simulink model "may9js"  (R2015a)
settings: Solver=ode4  StartTime=0.0  StopTime=inf  FixedStep=BKIN_STEP_TIME  RelTol=1e-3
StartFcn:
  |  warndlg('Dexterit-E models cannot run under simulation. Please compile your model and run it from within Dexterit-E.');set_param(bdroot,'SimulationCommand','stop')
model workspace (MAT data in the model file):
  BARRIER_ROW = 5
  BKIN_KINEMATIC_FRAME_SIZE = 400
  BKIN_STEP_TIME = 0.00025
  CIRCLE_ROW = 2
  CIRCLE_STROKE = 10
  CIRCLE_STROKE_W = 11
  E_BARRIER_HIT = 6
  E_COLLISION_HIT = 7
  E_ENTER_PRESHOT_AREA = 2
  E_ENTER_START_AREA = 12
  E_EXIT = 13
  E_EXIT_PRESHOT_AREA = 10
  E_GOAL_HIT = 8
  E_GOAL_REACHED = 5
  E_NO_EVENT = 0
  E_PRESHOT_ROW = 4
  E_TARGET_OUT_OF_BOUNDS = 9
  E_TRIAL_BEGIN = 1
  E_TRIAL_ENDED = 3
  FIRST_STATE_FILL = 9
  FORCE_MULTIPLIER = 1
  F_BUMP = 1
  GOAL_ROW = 8
  GOAL_TIME = 15
  HEIGHT = 6
  INVISIBLE_FILL = 15
  LOAD_ROW = 4
  MASS_BARRIER = 6
  MASS_CIRCLE = 2
  MASS_RECT = 3
  NEW_FLOAT = 10
  NEW_ROW = 9
  NEW_TEXTSIZE = 11
  PERT_DUR = 5
  PERT_RAMP = 4
  PRESHOT_ROW = 7
  RADIUS_LOG = 4
  RADIUS_VIS = 5
  RECT_FILL = 12
  RECT_ROW = 3
  RECT_STROKE = 13
  RECT_STROKE_W = 14
  ROTATION = 7
  SECONDS = 1
  SECOND_STATE_FILL = 8
  SHOT_READY_TIME = 13
  SHOT_SET_TIME = 14
  START_HOLD_TIME = 12
  START_ROW = 6
  TRIAL_FAILURE = 11
  WIDTH = 3
  col_x = 1
  col_y = 2
undefined symbols (not defined in the file): slselsubs
libraries: Video x7, General x3, KINARM_loads x2, KINARM_EP_loads x1, KINARM_general x1, simulink x1, slrtlib x1
(part 3 of 4)

== stateflow chart may9js/subsystem for moving the square (updating velocity and checking collision)/Collision Resolution ==
  settings: sampleTime=0.001
  state Initialize/
    % Stateflow starts here when task is loaded
    entry: force_scaling = [0 0 0 0];
    rect_target_out = zeros(1,70);
    rect_vel = [0 0];
    rect_offset_position = [0 0];
    trial_step = 0;
    trial_stop = 0;
  state Initialize1/
    % Stateflow starts here when task is loaded
    entry: force_scaling = [0 0 0 0];
    rect_target_out = zeros(1,70);
    rect_vel = [0 0];
    rect_offset_position = [0 0];
    trial_step = 0;
    trial_stop = 0;
  state Moving_Targets_and_Colliding_Them
    %there are 4 parallel states here. They each execute in the same cycle but in a specific order (see top right of the state)
    % state 3 is the important one - it simply says "move the square according to its velocity"
    % states 1 and 2 check collisions to update that velocity before we get to state 3
    % state 4 then checks to see if we ended up outside the screen and if so, to take us back to the start position
    state CollisionWithWall/ [parallel] [commented out]
      % this substate will handle collision between square and screen edges.
      % is the rectangle at the left edge of the screen
      en, du: if((rect_target_out(3)-rect_target_out(10)/2) < -display_size(1)/2)
      %rect_vel(1) = -rect_vel(1);
      trial_step = 2
      rect_vel(1) = 0;
      end
      % is the rectangle at the right edge of the screen
      if((rect_target_out(3)+rect_target_out(10)/2) > display_size(1)/2)
      %rect_vel(1) = -rect_vel(1);
      trial_step = 2
      rect_vel(1) = 0;
      end
      % is the rectangle at top of the scren
      if((rect_target_out(4)+rect_target_out(11)/2) > display_size(2))
      %rect_vel(2) = -rect_vel(2);
      trial_step = 2
      rect_vel(2) = 0;
      end
      % is the rectangle at bottom of the scren
      if((rect_target_out(4)-rect_target_out(11)/2) < 0)
      trial_step = 2
      rect_vel(2) = 0;
      %rect_vel(2) = -rect_vel(2);
      end
    state CheckToSeeIfWeAreOutofBounds1/ [parallel] [commented out]
      % once everything is done moving and colliding, we check to see if we're off the screen still. If we are, put the square in the start position with 0 velocity
      % once collision is handled, move the square by its velocity
      % Reset everything as soon as the rectangle touches the side of the screen
      during:
      if (rect_target_out(3) - rect_target_out(10)/2 <= -display_size(1)/2) || ...
      (rect_target_out(3) + rect_target_out(10)/2 >= display_size(1)/2) || ...
      (rect_target_out(4) + rect_target_out(11)/2 >= display_size(2)) || ...
      (rect_target_out(4) - rect_target_out(11)/2 <= 0)
      % Reset all movement variables
      rect_vel = [0, 0];  % Stop movement
      rect_offset_position = [0, 0];  % Reset position
      trial_step = 4;
      trial_stop = 1;  % Set flag to stop trial
      end
    state CheckToSeeIfGoalReached1/ [parallel] [commented out]
      % once the participant hits the square (denoted by the puck), then we want to calculate if it is inside of the goal or not. this is done using the input form prior matrix.
      % since the input ot this block is the vcode, we access the dimesnion of the vector that contains length., width, height. in the start position with 0 velocity
      % Get rectangle (puck) info
      rect_x = rect_target_out(3);
      rect_y = rect_target_out(4);
      rect_w = rect_target_out(10);
      rect_h = rect_target_out(11);
      % Get goal info
      goal_x = goal_target(3);
      goal_y = goal_target(4);
      goal_w = goal_target(10);
      goal_h = goal_target(11);
      % Compute edges
      rect_left   = rect_x - rect_w / 2;
      rect_right  = rect_x + rect_w / 2;
      rect_top    = rect_y + rect_h / 2;
      rect_bottom = rect_y - rect_h / 2;
      goal_left   = goal_x - goal_w / 2;
      goal_right  = goal_x + goal_w / 2;
      goal_top    = goal_y + goal_h / 2;
      goal_bottom = goal_y - goal_h / 2;
      % Check for full puck in goal (fully inside goal)
      if (rect_left >= goal_left) && (rect_right <= goal_right) && ...
      (rect_bottom >= goal_bottom) && (rect_top <= goal_top)
      % Fully inside goal
      trial_step = 3;
      trial_stop = 1;
      %rect_vel = [0, 0];  % Stop motion
      %rect_offset_position = [0, 0];  % Optionalreset
      end
    state CollisionWithHand/ [parallel]
      % this substate will handle collision checks between hands and the square
      settings: executionOrder=1
      state ResolveTargetCollision
        during: % if something collided, we're going to separate the two objects and then use elastic collision to update velocities
        % eject the rectangle
        rect_offset_position = eject( circ_target( target_colliding,:), rect_target, rect_offset_position);
        prev_vel = rect_vel;
        hand_vel = hand_speed( target_colliding,:)/1e3;
        % elastic collision equations - here m = 1 and is the same for hand and square. It is used here to provide relative mass
        % between the two objects. The forces here will be further multiplied by a fudge factor (see the Simulink forces section)
        rect_vel(1) = (mr - mc)/(mr + mc)*rect_vel(1) + 2*mc/(mc + mr)*hand_vel(1);
        rect_vel(2) = (mr - mc)/(mr + mc)*rect_vel(2) + 2*mc/(mc + mr)*hand_vel(2);
        hand_vector = [1 2; 3 4];
        % a bump will be generated that will be proportional to change in velocity
        force_scaling(hand_vector(target_colliding,:)) = prev_vel - rect_vel;
      state WaitForCollision/
        entry: % state where we wait for collisions to happen
        force_scaling = [0 0 0 0];
        during:
        rect_target_out = rect_target;
        rect_offset_position = rect_offset_position + rect_vel;
        rect_target_out(3:4) = rect_target_out(3:4)+rect_offset_position
        target_colliding = check_collision(circ_target, rect_target, rect_offset_position)
      state StartWithSpeed0/
        %
        entry:  rect_vel = [0 0];
        rect_offset_position = [0 0];
      Moving_Targets_and_Colliding_Them.CollisionWithHand.WaitForCollision -> Moving_Targets_and_Colliding_Them.CollisionWithHand.StartWithSpeed0 [order 2] : e_Trial_Start
      Moving_Targets_and_Colliding_Them.CollisionWithHand.StartWithSpeed0 -> Moving_Targets_and_Colliding_Them.CollisionWithHand.WaitForCollision
      Moving_Targets_and_Colliding_Them.CollisionWithHand.WaitForCollision -> Moving_Targets_and_Colliding_Them.CollisionWithHand.ResolveTargetCollision [order 1] : [ target_colliding]
      Moving_Targets_and_Colliding_Them.CollisionWithHand.ResolveTargetCollision -> Moving_Targets_and_Colliding_Them.CollisionWithHand.WaitForCollision : [~check_collision(circ_target( target_colliding,:), rect_target, rect_offset_position)]
          | /{target_colliding=0}
    state PositionUpdated/ [parallel]
      % once collision is handled, move the square by its velocity
      during: rect_target_out = rect_target;
      rect_offset_position = rect_offset_position + rect_vel;
      rect_target_out(3:4) = rect_target_out(3:4)+rect_offset_position;
      settings: executionOrder=2
  state Moving_Targets_and_Colliding_Them1
    %there are 4 parallel states here. They each execute in the same cycle but in a specific order (see top right of the state)
    % state 3 is the important one - it simply says "move the square according to its velocity"
    % states 1 and 2 check collisions to update that velocity before we get to state 3
    % state 4 then checks to see if we ended up outside the screen and if so, to take us back to the start position
    state PositionUpdated/ [parallel]
      % once collision is handled, move the square by its velocity
      during: rect_target_out = rect_target;
      rect_offset_position = rect_offset_position + rect_vel;
      rect_target_out(3:4) = rect_target_out(3:4)+rect_offset_position;
      settings: executionOrder=2
    state CollisionWithHand/ [parallel]
      % this substate will handle collision checks between hands and the square
      settings: executionOrder=1
      state StartWithSpeed0/
        %
        entry:  rect_vel = [0 0];
        rect_offset_position = [0 0];
      state WaitForCollision/
        entry: % state where we wait for collisions to happen
        force_scaling = [0 0 0 0];
        during:
        rect_target_out = rect_target;
        rect_offset_position = rect_offset_position + rect_vel;
        rect_target_out(3:4) = rect_target_out(3:4)+rect_offset_position
        target_colliding = check_collision(circ_target, rect_target, rect_offset_position)
      state ResolveTargetCollision
        during: % if something collided, we're going to separate the two objects and then use elastic collision to update velocities
        % eject the rectangle
        rect_offset_position = eject( circ_target( target_colliding,:), rect_target, rect_offset_position);
        prev_vel = rect_vel;
        hand_vel = hand_speed( target_colliding,:)/1e3;
        % elastic collision equations - here m = 1 and is the same for hand and square. It is used here to provide relative mass
        % between the two objects. The forces here will be further multiplied by a fudge factor (see the Simulink forces section)
        rect_vel(1) = (mr - mc)/(mr + mc)*rect_vel(1) + 2*mc/(mc + mr)*hand_vel(1);
        rect_vel(2) = (mr - mc)/(mr + mc)*rect_vel(2) + 2*mc/(mc + mr)*hand_vel(2);
        hand_vector = [1 2; 3 4];
        % a bump will be generated that will be proportional to change in velocity
        force_scaling(hand_vector(target_colliding,:)) = prev_vel - rect_vel;
      Moving_Targets_and_Colliding_Them1.CollisionWithHand.WaitForCollision -> Moving_Targets_and_Colliding_Them1.CollisionWithHand.StartWithSpeed0 [order 2] : e_Trial_Start
      Moving_Targets_and_Colliding_Them1.CollisionWithHand.StartWithSpeed0 -> Moving_Targets_and_Colliding_Them1.CollisionWithHand.WaitForCollision
      Moving_Targets_and_Colliding_Them1.CollisionWithHand.WaitForCollision -> Moving_Targets_and_Colliding_Them1.CollisionWithHand.ResolveTargetCollision [order 1] : [ target_colliding]
      Moving_Targets_and_Colliding_Them1.CollisionWithHand.ResolveTargetCollision -> Moving_Targets_and_Colliding_Them1.CollisionWithHand.WaitForCollision : [~check_collision(circ_target( target_colliding,:), rect_target, rect_offset_position)]
          | /{target_colliding=0}
    state CheckToSeeIfGoalReached1/ [parallel] [commented out]
      % once the participant hits the square (denoted by the puck), then we want to calculate if it is inside of the goal or not. this is done using the input form prior matrix.
      % since the input ot this block is the vcode, we access the dimesnion of the vector that contains length., width, height. in the start position with 0 velocity
      % Get rectangle (puck) info
      rect_x = rect_target_out(3);
      rect_y = rect_target_out(4);
      rect_w = rect_target_out(10);
      rect_h = rect_target_out(11);
      % Get goal info
      goal_x = goal_target(3);
      goal_y = goal_target(4);
      goal_w = goal_target(10);
      goal_h = goal_target(11);
      % Compute edges
      rect_left   = rect_x - rect_w / 2;
      rect_right  = rect_x + rect_w / 2;
      rect_top    = rect_y + rect_h / 2;
      rect_bottom = rect_y - rect_h / 2;
      goal_left   = goal_x - goal_w / 2;
      goal_right  = goal_x + goal_w / 2;
      goal_top    = goal_y + goal_h / 2;
      goal_bottom = goal_y - goal_h / 2;
      % Check for full puck in goal (fully inside goal)
      if (rect_left >= goal_left) && (rect_right <= goal_right) && ...
      (rect_bottom >= goal_bottom) && (rect_top <= goal_top)
      % Fully inside goal
      trial_step = 3;
      trial_stop = 1;
      %rect_vel = [0, 0];  % Stop motion
      %rect_offset_position = [0, 0];  % Optionalreset
      end
    state CheckToSeeIfWeAreOutofBounds1/ [parallel] [commented out]
      % once everything is done moving and colliding, we check to see if we're off the screen still. If we are, put the square in the start position with 0 velocity
      % once collision is handled, move the square by its velocity
      % Reset everything as soon as the rectangle touches the side of the screen
      during:
      if (rect_target_out(3) - rect_target_out(10)/2 <= -display_size(1)/2) || ...
      (rect_target_out(3) + rect_target_out(10)/2 >= display_size(1)/2) || ...
      (rect_target_out(4) + rect_target_out(11)/2 >= display_size(2)) || ...
      (rect_target_out(4) - rect_target_out(11)/2 <= 0)
      % Reset all movement variables
      rect_vel = [0, 0];  % Stop movement
      rect_offset_position = [0, 0];  % Reset position
      trial_step = 4;
      trial_stop = 1;  % Set flag to stop trial
      end
    state CollisionWithWall/ [parallel] [commented out]
      % this substate will handle collision between square and screen edges.
      % is the rectangle at the left edge of the screen
      en, du: if((rect_target_out(3)-rect_target_out(10)/2) < -display_size(1)/2)
      %rect_vel(1) = -rect_vel(1);
      trial_step = 2
      rect_vel(1) = 0;
      end
      % is the rectangle at the right edge of the screen
      if((rect_target_out(3)+rect_target_out(10)/2) > display_size(1)/2)
      %rect_vel(1) = -rect_vel(1);
      trial_step = 2
      rect_vel(1) = 0;
      end
      % is the rectangle at top of the scren
      if((rect_target_out(4)+rect_target_out(11)/2) > display_size(2))
      %rect_vel(2) = -rect_vel(2);
      trial_step = 2
      rect_vel(2) = 0;
      end
      % is the rectangle at bottom of the scren
      if((rect_target_out(4)-rect_target_out(11)/2) < 0)
      trial_step = 2
      rect_vel(2) = 0;
      %rect_vel(2) = -rect_vel(2);
      end
  (default) -> Initialize
  Initialize -> Moving_Targets_and_Colliding_Them.CollisionWithHand.StartWithSpeed0
  data: colliding_target function_output; circ_matrix_in function_input; rect_vector_in function_input; rect_offset_in function_input; colliding_target function_output; circ_matrix_in function_input; rect_vector_in function_input; rect_offset_in function_input; eject_rect_offset function_output; circ_vcode_in function_input; rect_vcode_in function_input; rect_offset function_input; eject_rect_offset function_output; circ_vcode_in function_input; rect_vcode_in function_input; rect_offset function_input; trial_protocol input; circ_target input double; circ_to_barrier_target input; rect_target_out output size=[1 70]; rect_target input; barrier_target input size=[1 70]; display_size input; force_scaling output; mc input; mr input; hand_vector local; rect_vel local; prev_vel local; target_colliding local; hand_vel local; rect_offset_position local double; trial_stop output double size=[1]; goal_target input; trial_step output; mb input size=1; barrier_colliding local; hand_speed input; check_collision_barrier1 local; barrier_vel local; force_scaling_barrier local; rect_y local; rect_w local; rect_h local; rect_x local; goal_h local; goal_y local; goal_w local; goal_x local; rect_top local; goal_top local; hand_offset_position local; prev_hand_vel local; rect_left local; rect_bottom local; goal_right local; rect_right local; goal_bottom local; goal_left local; new_hand_posistion_c local
  events: e_clk input RISING_EDGE_EVENT; e_Trial_Start input EITHER_EDGE_EVENT; e_Trial_Start1 input EITHER_EDGE_EVENT
  function colliding_target = check_collision(circ_matrix_in, rect_vector_in, rect_offset_in):
    | function colliding_target = check_collision(circ_matrix_in, rect_vector_in, rect_offset_in)
    | 
    | % calculates collision between 2 circles (ie. either hand feedback) and rectangle
    | % inputs:
    | %        circ_matrix_in - 2x70 matrix that is 2 circle vcodes
    | %        rect_vector_in - 1x70 vector that is a rectangle vcode
    | %        rect_offset_in - position offset for rect_vector_ in to calculate
    | %                         where the rectangle is
    | % outputs:
    | %        colliding_target values:
    | %              0- if nothing colliding
    | %              1- if rectangle collided with right hand
    | %              2- if rectangle colliding with left hand
    | 
    | x = 3;
    | y = 4;
    | 
    | colliding_target = 0;
    | 
    | for ii = 1:size(circ_matrix_in,1)
    | 	
    | 	current_circle_vcode = circ_matrix_in(ii,:);
    | 	
    | 	radius = current_circle_vcode(10);
    | 	w = rect_vector_in(10);
    | 	h = rect_vector_in(10);
    | 	
    | 	x0 = current_circle_vcode(x);
    | 	y0 = current_circle_vcode(y);
    | 	
    | 	X0 = rect_vector_in(x)+rect_offset_in(1);
    | 	Y0 = rect_vector_in(y)+rect_offset_in(2);
    | 	
    | 	deltax = x0-X0;
    | 	deltay = y0-Y0;
    | 	
    | 	w = rect_vector_in(10);  %width (sizes in cm in v1.4)
    | 	h = rect_vector_in(11);  %height (sizes in cm in v1.4)
    | 	
    | 	t = rect_vector_in(12)/180*pi;
    | 	
    | 	sint=sin(t);
    | 	cost=cos(t);
    | 	
    | 	xrotate=deltax.*cost + deltay.*sint;   %location of x point in rectangle's coordinate frame
    | 	yrotate=-deltax.*sint + deltay.*cost;  %location of y point in rectangle's coordinate frame
    | 		
    | 	%intarget = (abs(xrotate) < (w/2+radius)) & (abs(yrotate) < (h/2+radius));
    | 	
    | 	%--------------%
    | 	DeltaX = xrotate - max(0 - w/2, min(xrotate, 0 + w/2));
    | 	DeltaY = yrotate - max(0 - h/2, min(yrotate, 0 + h/2));
    | 	intarget = 1*(DeltaX * DeltaX + DeltaY * DeltaY) < (radius * radius);
    | 	
    | 	%--------------%
    | 	
    | 	
    | 	if intarget
    | 		colliding_target = ii;
    | 		break;
    | 	end
    | 	
    | end
  function colliding_target = check_collision1(circ_matrix_in, rect_vector_in, rect_offset_in):
    | function colliding_target = check_collision1(circ_matrix_in, rect_vector_in, rect_offset_in)
    | 
    | % calculates collision between 2 circles (ie. either hand feedback) and rectangle
    | % inputs:
    | %        circ_matrix_in - 2x70 matrix that is 2 circle vcodes
    | %        rect_vector_in - 1x70 vector that is a rectangle vcode
    | %        rect_offset_in - position offset for rect_vector_ in to calculate
    | %                         where the rectangle is
    | % outputs:
    | %        colliding_target values:
    | %              0- if nothing colliding
    | %              1- if rectangle collided with right hand
    | %              2- if rectangle colliding with left hand
    | 
    | x = 3;
    | y = 4;
    | 
    | colliding_target = 0;
    | 
    | for ii = 1:size(circ_matrix_in,1)
    | 	
    | 	current_circle_vcode = circ_matrix_in(ii,:);
    | 	
    | 	radius = current_circle_vcode(10);
    | 	w = rect_vector_in(10);
    | 	h = rect_vector_in(10);
    | 	
    | 	x0 = current_circle_vcode(x);
    | 	y0 = current_circle_vcode(y);
    | 	
    | 	X0 = rect_vector_in(x)+rect_offset_in(1);
    | 	Y0 = rect_vector_in(y)+rect_offset_in(2);
    | 	
    | 	deltax = x0-X0;
    | 	deltay = y0-Y0;
    | 	
    | 	w = rect_vector_in(10);  %width (sizes in cm in v1.4)
    | 	h = rect_vector_in(11);  %height (sizes in cm in v1.4)
    | 	
    | 	t = rect_vector_in(12)/180*pi;
    | 	
    | 	sint=sin(t);
    | 	cost=cos(t);
    | 	
    | 	xrotate=deltax.*cost + deltay.*sint;   %location of x point in rectangle's coordinate frame
    | 	yrotate=-deltax.*sint + deltay.*cost;  %location of y point in rectangle's coordinate frame
    | 		
    | 	%intarget = (abs(xrotate) < (w/2+radius)) & (abs(yrotate) < (h/2+radius));
    | 	
    | 	%--------------%
    | 	DeltaX = xrotate - max(0 - w/2, min(xrotate, 0 + w/2));
    | 	DeltaY = yrotate - max(0 - h/2, min(yrotate, 0 + h/2));
    | 	intarget = 1*(DeltaX * DeltaX + DeltaY * DeltaY) < (radius * radius);
    | 	
    | 	%--------------%
    | 	
    | 	
    | 	if intarget
    | 		colliding_target = ii;
    | 		break;
    | 	end
    | 	
    | end
  function eject_rect_offset = eject(circ_vcode_in, rect_vcode_in, rect_offset):
    | function eject_rect_offset = eject(circ_vcode_in, rect_vcode_in, rect_offset)
    | 
    | % moves the rectangle_vcode out of a circle_vcode if the two are
    | % overlapping
    | 
    | x = 3;
    | y = 4;
    | 
    | radius = circ_vcode_in(10);
    | w = rect_vcode_in(10);
    | h = rect_vcode_in(10);
    | 
    | x0 = circ_vcode_in(x);
    | y0 = circ_vcode_in(y);
    | 
    | X0 = rect_vcode_in(x)+rect_offset(1);
    | Y0 = rect_vcode_in(y)+rect_offset(2);
    | 
    | deltax = x0-X0;
    | deltay = y0-Y0;
    | 
    | w = rect_vcode_in(10);  %width (sizes in cm in v1.4)
    | h = rect_vcode_in(11);  %height (sizes in cm in v1.4)
    | 
    | t = rect_vcode_in(12)/180*pi;
    | 
    | sint=sin(t);
    | cost=cos(t);
    | 
    | xrotate=deltax.*cost + deltay.*sint;   %location of x point in rectangle's coordinate frame
    | yrotate=-deltax.*sint + deltay.*cost;  %location of y point in rectangle's coordinate frame
    | 
    | % so xrotate and yrotate is where the circle is inside the rectangle
    | theta_threshold = atan(h / w); % get the threshold - angles below this go out the side while angles
    | % above this go out the top
    | 
    | % calculating magnitude
    | 
    | % polar coordinate to the circle
    | [t_c, ~] = cart2pol(abs(xrotate), abs(yrotate));
    | 
    | if t_c < theta_threshold % the rectangle will be moved along its local x-axis to exit the circle
    |     x_eject_local = (w/2+radius-abs(xrotate))*sign(-xrotate); % if the circle is on the right, move the rectangle left and vice-versa
    |     y_eject_local = 0;
    | else % going out top/bottom % the rectangle will be moved along its local y-axis to exit the circle
    |     x_eject_local = 0;
    |     y_eject_local = (h/2+radius-abs(yrotate))*sign(-yrotate); % if the circle is above the rectangle, move the rectangle down and vice-versa
    | end
    | 
    | % convert the local offsets to global coordinates by undoing the rotation
    | 
    | % rotate back to global coordinates
    | sint=sin(-t);
    | cost=cos(-t);
    | 
    | x_eject_global = x_eject_local.*cost + y_eject_local.*sint;   
    | y_eject_global = - x_eject_local.*sint + y_eject_local.*cost;
    | 
    | eject_rect_offset = rect_offset + [x_eject_global y_eject_global];
  function eject_rect_offset = eject1(circ_vcode_in, rect_vcode_in, rect_offset):
    | function eject_rect_offset = eject1(circ_vcode_in, rect_vcode_in, rect_offset)
    | 
    | % moves the rectangle_vcode out of a circle_vcode if the two are
    | % overlapping
    | 
    | x = 3;
    | y = 4;
    | 
    | radius = circ_vcode_in(10);
    | w = rect_vcode_in(10);
    | h = rect_vcode_in(10);
    | 
    | x0 = circ_vcode_in(x);
    | y0 = circ_vcode_in(y);
    | 
    | X0 = rect_vcode_in(x)+rect_offset(1);
    | Y0 = rect_vcode_in(y)+rect_offset(2);
    | 
    | deltax = x0-X0;
    | deltay = y0-Y0;
    | 
    | w = rect_vcode_in(10);  %width (sizes in cm in v1.4)
    | h = rect_vcode_in(11);  %height (sizes in cm in v1.4)
    | 
    | t = rect_vcode_in(12)/180*pi;
    | 
    | sint=sin(t);
    | cost=cos(t);
    | 
    | xrotate=deltax.*cost + deltay.*sint;   %location of x point in rectangle's coordinate frame
    | yrotate=-deltax.*sint + deltay.*cost;  %location of y point in rectangle's coordinate frame
    | 
    | % so xrotate and yrotate is where the circle is inside the rectangle
    | theta_threshold = atan(h / w); % get the threshold - angles below this go out the side while angles
    | % above this go out the top
    | 
    | % calculating magnitude
    | 
    | % polar coordinate to the circle
    | [t_c, ~] = cart2pol(abs(xrotate), abs(yrotate));
    | 
    | if t_c < theta_threshold % the rectangle will be moved along its local x-axis to exit the circle
    |     x_eject_local = (w/2+radius-abs(xrotate))*sign(-xrotate); % if the circle is on the right, move the rectangle left and vice-versa
    |     y_eject_local = 0;
    | else % going out top/bottom % the rectangle will be moved along its local y-axis to exit the circle
    |     x_eject_local = 0;
    |     y_eject_local = (h/2+radius-abs(yrotate))*sign(-yrotate); % if the circle is above the rectangle, move the rectangle down and vice-versa
    | end
    | 
    | % convert the local offsets to global coordinates by undoing the rotation
    | 
    | % rotate back to global coordinates
    | sint=sin(-t);
    | cost=cos(-t);
    | 
    | x_eject_global = x_eject_local.*cost + y_eject_local.*sint;   
    | y_eject_global = - x_eject_local.*sint + y_eject_local.*cost;
    | 
    | eject_rect_offset = rect_offset + [x_eject_global y_eject_global];

== matlab function may9js/subsystem for moving the square (updating velocity and checking collision)/Hand Feedback/MATLAB Function ==
  data: feedback_vcodes input; arm_to_be_assessed input; hand_vcodes output
function hand_vcodes = fcn(feedback_vcodes, arm_to_be_assessed)
% the hand feedback vcodes are sorted like this:
%    <arm to be assessed vcode>
%    <contralateral arm> 
% but using this function I am going to sort the vcodes like this:
%    <right arm>
%    <left arm>
% because that will make it easier to track velocities and forces

if arm_to_be_assessed == 1
	hand_vcodes = feedback_vcodes;
else
	hand_vcodes = feedback_vcodes([2 1], :);
	%hand_vcodes = feedback_vcodes;
end

== stateflow chart may9js/Trial_Control ==
  settings: sampleTime=0.001
  state Initialize/
    % Set variables
    entry:
    logging_enable = true;
    start_target_row = Trial_Protocol(START_ROW);
    preshot_area_row = Trial_Protocol(PRESHOT_ROW);
    cursor_row = Trial_Protocol(CIRCLE_ROW);
    puck_row = Trial_Protocol(RECT_ROW);
    barrier_target_row = Trial_Protocol(BARRIER_ROW);
    goal_target_row = Trial_Protocol(GOAL_ROW);
    load_row = Trial_Protocol(LOAD_ROW);
    trial_duration = Trial_Protocol(SECONDS);
    start_hold_time = Trial_Protocol(START_HOLD_TIME);
    shot_ready_time = Trial_Protocol(SHOT_READY_TIME);
    shot_set_time = Trial_Protocol(SHOT_SET_TIME);
    goal_time = Trial_Protocol(GOAL_TIME);
  state Main_Trial/
    % Each trial task only initializes variables and then runs for Trial_Protocol(SECONDS) seconds before stopping
    state StartOn/
      entry:
      start_target_state = 2;
      preshot_area_state = 0;
      cursor_state = 2;
      puck_state = 0;
      barrier_target_state = 0;
      goal_target_state = 0;
      e_Trial_Start;
      event_code = E_TRIAL_BEGIN;
    state StartHold/
      entry:
      start_target_state = 3;
      preshot_area_state=0;
      puck_state=0;
      goal_target_state=0;
      barrier_target_state=0;
      event_code = E_ENTER_START_AREA;
    state PreshotStart/
      % send e_Trial_End event
      entry:
      preshot_area_state=3;
      puck_state=2;
      goal_target_state=2;
      barrier_target_state=2;
      event_code = E_ENTER_PRESHOT_AREA;
    state PreshotMove/
      % send e_Trial_End event
      entry:
    state CollisionWithHand/
      % this substate will handle collision checks between hands and the square
      state StartWithSpeed0/
        %
        entry:  rect_vel = [0 0];
        rect_offset_position = [0 0];
      state WaitForCollision/
        entry: % state where we wait for collisions to happen
        force_scaling = [0 0 0 0];
        during:
        rect_target_out = rect_target;
        rect_offset_position = rect_offset_position + rect_vel;
        rect_target_out(3:4) = rect_target_out(3:4)+rect_offset_position
        target_colliding = check_collision(circ_target, rect_target, rect_offset_position)
      state ResolveTargetCollision
        during: % if something collided, we're going to separate the two objects and then use elastic collision to update velocities
        % eject the rectangle
        rect_offset_position = eject( circ_target( target_colliding,:), rect_target, rect_offset_position);
        prev_vel = rect_vel;
        hand_vel = hand_speed( target_colliding,:)/1e3;
        % elastic collision equations - here m = 1 and is the same for hand and square. It is used here to provide relative mass
        % between the two objects. The forces here will be further multiplied by a fudge factor (see the Simulink forces section)
        rect_vel(1) = (mr - mc)/(mr + mc)*rect_vel(1) + 2*mc/(mc + mr)*hand_vel(1);
        rect_vel(2) = (mr - mc)/(mr + mc)*rect_vel(2) + 2*mc/(mc + mr)*hand_vel(2);
        hand_vector = [1 2; 3 4];
        % a bump will be generated that will be proportional to change in velocity
        force_scaling(hand_vector(target_colliding,:)) = prev_vel - rect_vel;
      WaitForCollision -> StartWithSpeed0 [order 2] : e_Trial_Start
      StartWithSpeed0 -> WaitForCollision
      WaitForCollision -> ResolveTargetCollision [order 1] : [ target_colliding]
      ResolveTargetCollision -> WaitForCollision : [~check_collision(circ_target( target_colliding,:), rect_target, rect_offset_position)]
          | /{target_colliding=0}
    state ShotReady/
      % send e_Trial_End event
      entry:
      event_code = E_EXIT;
    state ShotSet/
      % send e_Trial_End event
      entry:
      preshot_area_state=0;
    state Success/
      % send e_Trial_End event
      entry:
      puck_state=0;
      goal_target_state=3
    state PuckInGoal/
      % send e_Trial_End event
      entry:
    state Shot/
      % send e_Trial_End event
      entry:
      start_target_state=0;
    state Fail/
      % send e_Trial_End event
      entry:
      event_code = E_TRIAL_FAILURE;
      start_target_state=0;
      preshot_area_state = 0;
      cursor_state = 2;
      puck_state = 0;
      barrier_target_state = 0;
      goal_target_state = 0;
    state PositionUpdated/
      % once collision is handled, move the square by its velocity
      during: rect_target_out = rect_target;
      rect_offset_position = rect_offset_position + rect_vel;
      rect_target_out(3:4) = rect_target_out(3:4)+rect_offset_position;
    state Initialize1/
      % Stateflow starts here when task is loaded
      entry: force_scaling = [0 0 0 0];
      rect_target_out = zeros(1,70);
      rect_vel = [0 0];
      rect_offset_position = [0 0];
      trial_step = 0;
      trial_stop = 0;
    StartHold -> PreshotStart [order 2] : after(start_hold_time,sec)
    StartOn -> StartHold [order 1] : [HandInTarget(start_target_row,1)==1]
    StartHold -> StartOn [order 1] : [HandInTarget(start_target_row,1)==0]
    PreshotStart -> PreshotMove [order 2] : [HandInTarget(start_target_row,1)==0]
    PreshotStart -> StartHold [order 1] : [HandInTarget(preshot_area_row,1)==0]
    ShotSet -> StartOn [order 1] : [HandInTarget(start_target_row,1)==0]
    PreshotMove -> StartOn [order 2] : [HandInTarget(preshot_area_row,1)==0]
    ShotReady -> PreshotMove [order 1] : [HandInTarget(start_target_row,1)==0]
    PreshotMove -> ShotReady [order 1] : [HandInTarget(start_target_row,1)==1]
    ShotReady -> StartWithSpeed0 [order 2]
    ShotReady -> ShotSet [order 3] : after(shot_ready_time,sec)
    ShotSet -> Shot [order 2] : after(shot_set_time,sec)
    PuckInGoal -> Success [order 1] : after(goal_time,sec)
    Shot -> PuckInGoal [order 3] : [PuckInTarget(goal_target_row,1)==1]
    PuckInGoal -> Fail [order 2] : [PuckInTarget(goal_target_row,1)==0]
    Shot -> Fail [order 2] : [HandInBarrier(barrier_target_row,1)==1]
    Shot -> Fail [order 1] : after(trial_duration,sec)
  state Inter_Trial_State/
    % send e_Trial_End event
    entry:
    e_Trial_End;
    event_code = E_TRIAL_ENDED;
  state CollisionWithWall/ [commented out]
    % this substate will handle collision between square and screen edges.
    % is the rectangle at the left edge of the screen
    en, du: if((rect_target_out(3)-rect_target_out(10)/2) < -display_size(1)/2)
    %rect_vel(1) = -rect_vel(1);
    trial_step = 2
    rect_vel(1) = 0;
    end
    % is the rectangle at the right edge of the screen
    if((rect_target_out(3)+rect_target_out(10)/2) > display_size(1)/2)
    %rect_vel(1) = -rect_vel(1);
    trial_step = 2
    rect_vel(1) = 0;
    end
    % is the rectangle at top of the scren
    if((rect_target_out(4)+rect_target_out(11)/2) > display_size(2))
    %rect_vel(2) = -rect_vel(2);
    trial_step = 2
    rect_vel(2) = 0;
    end
    % is the rectangle at bottom of the scren
    if((rect_target_out(4)-rect_target_out(11)/2) < 0)
    trial_step = 2
    rect_vel(2) = 0;
    %rect_vel(2) = -rect_vel(2);
    end
  (default) -> Initialize
  Initialize -> StartOn
  Inter_Trial_State -> StartOn : after(1, sec)
  StartOn -> Inter_Trial_State [order 2] : after(trial_duration, sec)
  Main_Trial -> Inter_Trial_State : e_ExitTrialNow
  Fail -> Inter_Trial_State : after(0.3,sec)
  Success -> Inter_Trial_State : after(0.3,sec)
  data: colliding_target function_output; circ_matrix_in function_input; rect_vector_in function_input; rect_offset_in function_input; eject_rect_offset function_output; circ_vcode_in function_input; rect_vcode_in function_input; rect_offset function_input; logging_enable output boolean; event_code output; cursor_row output; cursor_state output; puck_row output; puck_state output; load_row output; Trial_Protocol input; trial_duration local; barrier_target_row output; barrier_target_state output; start_target_row output; start_target_state output; goal_target_row output; goal_target_state output; HandInTarget input double; trial_ended input; trial_step_datas input; preshot_area_state output; preshot_area_row output; start_hold_time local; shot_set_time local; shot_ready_time local; HandInBarrier input double; PuckInTarget input; goal_time local; vcode_barrier input; vcode_preshot_area local; vcode_puck input; vcode_goal input; vcode_start input; vcode_hands input; data local; displaysize input; hand_speed input; mass_hand input; mass_rectangle input; mass_barrier input; puck_vcode_out output
  events: e_clk input RISING_EDGE_EVENT; e_ExitTrialNow input EITHER_EDGE_EVENT; e_Trial_End output EITHER_EDGE_EVENT; e_Trial_Start output EITHER_EDGE_EVENT
  function colliding_target = check_collision1(circ_matrix_in, rect_vector_in, rect_offset_in):
    | function colliding_target = check_collision1(circ_matrix_in, rect_vector_in, rect_offset_in)
    | 
    | % calculates collision between 2 circles (ie. either hand feedback) and rectangle
    | % inputs:
    | %        circ_matrix_in - 2x70 matrix that is 2 circle vcodes
    | %        rect_vector_in - 1x70 vector that is a rectangle vcode
    | %        rect_offset_in - position offset for rect_vector_ in to calculate
    | %                         where the rectangle is
    | % outputs:
    | %        colliding_target values:
    | %              0- if nothing colliding
    | %              1- if rectangle collided with right hand
    | %              2- if rectangle colliding with left hand
    | 
    | x = 3;
    | y = 4;
    | 
    | colliding_target = 0;
    | 
    | for ii = 1:size(circ_matrix_in,1)
    | 	
    | 	current_circle_vcode = circ_matrix_in(ii,:);
    | 	
    | 	radius = current_circle_vcode(10);
    | 	w = rect_vector_in(10);
    | 	h = rect_vector_in(10);
    | 	
    | 	x0 = current_circle_vcode(x);
    | 	y0 = current_circle_vcode(y);
    | 	
    | 	X0 = rect_vector_in(x)+rect_offset_in(1);
    | 	Y0 = rect_vector_in(y)+rect_offset_in(2);
    | 	
    | 	deltax = x0-X0;
    | 	deltay = y0-Y0;
    | 	
    | 	w = rect_vector_in(10);  %width (sizes in cm in v1.4)
    | 	h = rect_vector_in(11);  %height (sizes in cm in v1.4)
    | 	
    | 	t = rect_vector_in(12)/180*pi;
    | 	
    | 	sint=sin(t);
    | 	cost=cos(t);
    | 	
    | 	xrotate=deltax.*cost + deltay.*sint;   %location of x point in rectangle's coordinate frame
    | 	yrotate=-deltax.*sint + deltay.*cost;  %location of y point in rectangle's coordinate frame
    | 		
    | 	%intarget = (abs(xrotate) < (w/2+radius)) & (abs(yrotate) < (h/2+radius));
    | 	
    | 	%--------------%
    | 	DeltaX = xrotate - max(0 - w/2, min(xrotate, 0 + w/2));
    | 	DeltaY = yrotate - max(0 - h/2, min(yrotate, 0 + h/2));
    | 	intarget = 1*(DeltaX * DeltaX + DeltaY * DeltaY) < (radius * radius);
    | 	
    | 	%--------------%
    | 	
    | 	
    | 	if intarget
    | 		colliding_target = ii;
    | 		break;
    | 	end
    | 	
    | end
  function eject_rect_offset = eject1(circ_vcode_in, rect_vcode_in, rect_offset):
    | function eject_rect_offset = eject1(circ_vcode_in, rect_vcode_in, rect_offset)
    | 
    | % moves the rectangle_vcode out of a circle_vcode if the two are
    | % overlapping
    | 
    | x = 3;
    | y = 4;
    | 
    | radius = circ_vcode_in(10);
    | w = rect_vcode_in(10);
    | h = rect_vcode_in(10);
    | 
    | x0 = circ_vcode_in(x);
    | y0 = circ_vcode_in(y);
    | 
    | X0 = rect_vcode_in(x)+rect_offset(1);
    | Y0 = rect_vcode_in(y)+rect_offset(2);
    | 
    | deltax = x0-X0;
    | deltay = y0-Y0;
    | 
    | w = rect_vcode_in(10);  %width (sizes in cm in v1.4)
    | h = rect_vcode_in(11);  %height (sizes in cm in v1.4)
    | 
    | t = rect_vcode_in(12)/180*pi;
    | 
    | sint=sin(t);
    | cost=cos(t);
    | 
    | xrotate=deltax.*cost + deltay.*sint;   %location of x point in rectangle's coordinate frame
    | yrotate=-deltax.*sint + deltay.*cost;  %location of y point in rectangle's coordinate frame
    | 
    | % so xrotate and yrotate is where the circle is inside the rectangle
    | theta_threshold = atan(h / w); % get the threshold - angles below this go out the side while angles
    | % above this go out the top
    | 
    | % calculating magnitude
    | 
    | % polar coordinate to the circle
    | [t_c, ~] = cart2pol(abs(xrotate), abs(yrotate));
    | 
    | if t_c < theta_threshold % the rectangle will be moved along its local x-axis to exit the circle
    |     x_eject_local = (w/2+radius-abs(xrotate))*sign(-xrotate); % if the circle is on the right, move the rectangle left and vice-versa
    |     y_eject_local = 0;
    | else % going out top/bottom % the rectangle will be moved along its local y-axis to exit the circle
    |     x_eject_local = 0;
    |     y_eject_local = (h/2+radius-abs(yrotate))*sign(-yrotate); % if the circle is above the rectangle, move the rectangle down and vice-versa
    | end
    | 
    | % convert the local offsets to global coordinates by undoing the rotation
    | 
    | % rotate back to global coordinates
    | sint=sin(-t);
    | cost=cos(-t);
    | 
    | x_eject_global = x_eject_local.*cost + y_eject_local.*sint;   
    | y_eject_global = - x_eject_local.*sint + y_eject_local.*cost;
    | 
    | eject_rect_offset = rect_offset + [x_eject_global y_eject_global];

== matlab function may9js/subsystem for moving the square (updating velocity and checking collision)/Hand Feedback/Hand_Feedback/FeedFwdArm ==
  settings: fimath=|
      | fimath(...
      | 'RoundMode', 'floor',...
      | 'OverflowMode', 'wrap',...
      | 'ProductMode', 'KeepLSB', 'ProductWordLength', 32,...
      | 'SumMode', 'KeepLSB', 'SumWordLength', 32,...
      | 'CastBeforeSum', false)
  data: KINARMdata input; VCODES_in input; VCODES_out output; fdbk_stts_mdl input; block_settings input
function VCODES_out  = fcn(KINARMdata,VCODES_in,fdbk_stts_mdl, block_settings)
%
% This function creates the VCODEs for the hand position feedback for both
% hands.  Various options in the Mask of the Simulink block in which this
% embedded Matlab file sits, allow the user to specify how often
% the hand feedback is updated as well as the source of the style and status
% of the hand feedback.  
%
% block_settings is the value chosen by the user in the Mask for parent Simulink
% block.  Note: that even if the block is wired up to accept Task Program 
% control of hand feedback style and status, this embedded Matlab file allows
% the GUI to over-ride those settings.  However, if the GUI requests that
% the parent block use Task Program control for the style and/or status when
% it has not been programmed in, then this embedded Matlab file handles this
% appropriately and ignore the request for Task Program control.  
%
% block_settings=1 -- parent block does not have any Task Program control over style or status
% block_settings=2 -- parent block has Task Program control over status only
% block_settings=3 -- parent block has Task Program control over both style and status
%
% fdbk_stts_mdl (only potentially used if block_settings=2) 
% fdbk_stts_mdl=0 -- neither hand on
% fdbk_stts_mdl=1 -- dominant hand on
% fdbk_stts_mdl=2 -- non-dominant hand on
% fdbk_stts_mdl=3 -- both hands on
%
% VCODES (only potentially used if block_settings=3) 
% VCODES for dominant and non-dominant, input to parent block 


dominant_arm=KINARMdata(3,1);
feedfwd=KINARMdata(3,2);				%amount of feedforward extrapolation for hand position(s)
fdbk_stts_GUI=KINARMdata(3,3);			%status of hand feedback requested from GUI
fdbk_src_GUI=KINARMdata(3,4);			%source of hand feedback style requested from GUI
fdbk_clr_GUI=KINARMdata(3,5);			%colour of hand feedback required by GUI
fdbk_radius_GUI=KINARMdata(3,6);		%radius of hand feedback required by GUI


%----------------Feedback Style ----------------
% IF GUI asks for feedback style from Task Program (fdbk_src_GUI==0)
% AND if Task Program has been chosen to supply feedback style (block_settings==3)
% AND if Task Program actually supplies appropriate feedback styles (size(VCODES_in,2)==70)
if fdbk_src_GUI==0 && block_settings==3 && size(VCODES_in,2)==70
    VCODES=VCODES_in;
else
    VCODES=zeros(2,70);						%set default
	VCODES(:,1)=1;							%target_type of circle
	VCODES(:,5)=fdbk_clr_GUI;				%fill colour as specified by GUI
	VCODES(:,6)=fdbk_clr_GUI;				%stroke colour same as fill colour
	VCODES(:,7)=0;							%no stroke width
    VCODES(:,9)=100.0;                      %100% opacity
	VCODES(:,10)=fdbk_radius_GUI;			%radius (m) as specified by GUI
end

%----------------Feedback Status ----------------
%feedback status from GUI sets the default to be used
feedback_status=fdbk_stts_GUI;


if fdbk_stts_GUI==4				%if GUI has requested Task Program control of feedback status
	if block_settings==2		%if there is Task Program control ONLY of status (but not style)
		feedback_status=fdbk_stts_mdl;		%then use feedback status input from parent block
	elseif block_settings==3	%if there is Task Program control of both status and style
		feedback_status=4;		%then let the input VCODEs handle the status
	else						%otherwise assume that the Task Program did not provide style OR status
		feedback_status=3;		%then set both hands are always on as a default
    end
else		%if GUI is controlling feedback status
	feedback_status=fdbk_stts_GUI;
end

%set the status of the hand-feedback in the VCODES
switch feedback_status
	case 0					%show neither hand feedback
		VCODES(1,2)=0;
		VCODES(2,2)=0;
	case 1					%show ONLY dominant hand feedback
		VCODES(1,2)=1;
		VCODES(2,2)=0;
	case 2					%show ONLY non-dominant hand feedback
		VCODES(1,2)=0;
		VCODES(2,2)=1;
	case 4					%VCODES already control hand feedback
		%do nothing
	otherwise				%show both hand feedbacks
		VCODES(1,2)=1;
		VCODES(2,2)=1;
end

%----------------Feedback Position ----------------
%set the position of the hand feedback.
for i=1:2
	if i==1
		active_arm=KINARMdata(3,1);			%choose dominant arm first
	else
		active_arm=3-KINARMdata(3,1);		%choose non-dominant arm 2nd
	end
	HandXPos=KINARMdata(active_arm,23);		%(m)
	HandYPos=KINARMdata(active_arm,24);		%(m)
	HandXVel=KINARMdata(active_arm,25);		%(m/s)
	HandYVel=KINARMdata(active_arm,26);		%(m/s)

	% feed-forward hand position (m)
	%HandXPos_ff = HandXPos + HandXVel*feedfwd;
	%HandYPos_ff = HandYPos + HandYVel*feedfwd;
	HandXPos_ff = HandXPos;
	HandYPos_ff = HandYPos;
	VCODES(i,3)=HandXPos_ff;				%target position in m 
	VCODES(i,4)=HandYPos_ff;				%target position in m 
end

VCODES_out=VCODES;
